simulink model "UNIFIER1"  (R2023b)
settings: Solver=ode1  StartTime=0.0  StopTime=t_sim  FixedStep=1/500  RelTol=1e-3
values from neighbouring files (symbols this model uses):
  b = 20.11467    [UNIFIERLanding_20240613_190735.mat]    (also in UNIFIER_LOAD.m; UNIFIER_LOADsim.m; UNIFIER_trim_out_20240612_032607.mat)
  c = 1.43676    [UNIFIERLanding_20240613_190735.mat]    (also in UNIFIER_LOAD.m; UNIFIER_LOADsim.m; UNIFIER_trim_out_20240612_032607.mat)
  DEP_INTEG_IC = 117.49388    [UNIFIER_LOAD.m]    (also in UNIFIER_LOADsim.m; UNIFIER_trim_out_20240612_032607.mat)
  dp_DEP =     [UNIFIERLanding_20240613_190735.mat]    (also in UNIFIER_trim_out_20240612_032607.mat)
  dp_FUSE_FIN =     [UNIFIER_trim_out_20240612_032607.mat]
  dp_HTU =     [UNIFIERLanding_20240613_190735.mat]    (also in UNIFIER_trim_out_20240612_032607.mat)
  dp_VTAIL =     [UNIFIER_trim_out_20240612_032607.mat]
  dp_VTAIL_INDUCED =     [UNIFIER_trim_out_20240612_032607.mat]
  dp_WING_root =     [UNIFIER_trim_out_20240612_032607.mat]
  dp_WING_tip =     [UNIFIER_trim_out_20240612_032607.mat]
  dumax = [1.0471975512 1.0471975512 1.0471975512 0.174532925199 2 2 2]    [UNIFIERLanding_20240613_190735.mat]
  Euler0 = xstar(7:9)'    [UNIFIER_6DOFsim_init.m]    (also in UNIFIER_LOAD.m = [0, 0, 0]; UNIFIER_LOADsim.m; UNIFIER_trim_out_20240612_032607.mat = [3.43106170069e-06 0.0515008506278 -2.79252663434])
  ground_alt = 0    [UNIFIER_LOAD.m]    (also in UNIFIER_LOADsim.m; UNIFIER_trim_out_20240612_032607.mat)
  m = 7057    [UNIFIERLanding_20240613_190735.mat]    (also in UNIFIER_LOAD.m; UNIFIER_LOADsim.m; UNIFIER_trim_out_20240612_032607.mat)
  omegab0 = xstar(10:12)'    [UNIFIER_6DOFsim_init.m]    (also in UNIFIER_LOAD.m = [0,0,0]; UNIFIER_LOADsim.m; UNIFIER_trim_out_20240612_032607.mat = [0 0 0])
  S = 29.98388    [UNIFIERLanding_20240613_190735.mat]    (also in UNIFIER_LOAD.m; UNIFIER_LOADsim.m; UNIFIER_trim_out_20240612_032607.mat)
  sensor_delay_steps = 5    [UNIFIER_LOAD.m]    (also in UNIFIER_LOADsim.m; UNIFIER_trim_out_20240612_032607.mat)
  solution =     [UNIFIERLanding_20240613_190735.mat]
  u1_0 = [ustar(1), -1*ustar(1), ustar(3)-ustar(2), ustar(3)+ustar(2), ustar(4), ustar(4)]    [UNIFIER_6DOFsim_init.m]    (also in UNIFIER_LOAD.m = [2.1112539e-05, -2.1112539e-05, -0.085004635, -0.084972650, ; UNIFIER_LOADsim.m = [2.1112539e-05, -2.1112539e-05, -0.085004635, -0.084972650, ; UNIFIER_trim_out_20240612_032607.mat = [2.1112539e-05 -2.1112539e-05 -0.085004635 -0.08497265 0.197)
  u2_0 = ones(1,12) .* ustar(5)    [UNIFIER_6DOFsim_init.m]    (also in UNIFIER_LOAD.m = ones(1,12) .* 0.4252; UNIFIER_LOADsim.m = ones(1,12) .* 0.4252; UNIFIER_trim_out_20240612_032607.mat = [0.4252 0.4252 0.4252 0.4252 0.4252 0.4252 0.4252 0.4252 0.4)
  u3_0 = ustar(7)    [UNIFIER_6DOFsim_init.m]    (also in UNIFIER_LOAD.m = 0.089689; UNIFIER_LOADsim.m = 0.089689; UNIFIER_trim_out_20240612_032607.mat = 0.089689)
  u4_0 = 0    [UNIFIER_6DOFsim_init.m]    (also in UNIFIER_LOAD.m; UNIFIER_LOADsim.m; UNIFIER_trim_out_20240612_032607.mat)
  u_trim = ustar    [UNIFIER_6DOFsim_init.m]    (also in UNIFIER_LOAD.m = [0.0; UNIFIER_LOADsim.m)
  umax = [0.436332312999 0.523598775598 0.523598775598 0.436332312999 1 1 1]    [UNIFIERLanding_20240613_190735.mat]    (also in UNIFIER_trim_out_20240612_032607.mat)
  umin = [-0.436332312999 -0.523598775598 -0.523598775598 0 0 -1 -0.5]    [UNIFIERLanding_20240613_190735.mat]    (also in UNIFIER_trim_out_20240612_032607.mat)
  Va = [72.7399985115 72.2978466179 70.3592089076 68.5755686022 67.5674222915 66.8967003826 65.8958642605 64.4243196248 62.667507398 61.0171213882 59.8601734245 59.2796795419 ... (250 elements, 250x1)]    [UNIFIERLanding_20240613_190735.mat]
  Vb0 = xstar(4:6)'    [UNIFIER_6DOFsim_init.m]    (also in UNIFIER_LOAD.m = [72.731047032614440, 0, 1.142307104518741]; UNIFIER_LOADsim.m; UNIFIER_trim_out_20240612_032607.mat = [52.6789583502 0 2.71559652634])
  vtail_dist_to_wing = 7.8070    (= 7.807)    [UNIFIER_LOAD.m]    (also in UNIFIER_LOADsim.m; UNIFIER_trim_out_20240612_032607.mat)
  vtail_nodes = [dp_VTAIL.Xs_LE;     dp_VTAIL.Ys_LE;     dp_VTAIL.Zs_LE]    [UNIFIER_LOAD.m]    (also in UNIFIER_LOADsim.m; UNIFIER_trim_out_20240612_032607.mat = [-16.4894695282 -2.83441376686 -2.73765826225 -16.1370849609)
  wing_nodes = [fliplr(dp_WING_tip.LE_Xs),fliplr(dp_WING_root.LE_Xs),dp_WING_root.LE_Xs,dp_WING_tip.LE_Xs;     fliplr(-dp_WING_tip.LE_Ys),fliplr(-dp_WING_root.LE_Ys),dp_WING_root.LE_Ys,dp_WING_tip.LE_Ys;     fliplr(dp_WING_tip.LE_Zs),fliplr(dp_WING_root.LE_Zs),dp_WING_root.LE_Zs,dp_WING_tip.LE_Zs]    [UNIFIER_LOAD.m]    (also in UNIFIER_LOADsim.m; UNIFIER_trim_out_20240612_032607.mat = [-7.70795631409 -9.67500019073 -0.98178178072 -7.66801691055)
  Xe0 = xstar(1:3)'    [UNIFIER_6DOFsim_init.m]    (also in UNIFIER_LOAD.m = [0,0,-1219]; UNIFIER_LOADsim.m; UNIFIER_trim_out_20240612_032607.mat = [0 0 -1100])
  xyz_cg = [-8.09 0 -0.2]    [UNIFIERLanding_20240613_190735.mat]    (also in UNIFIER_LOAD.m = [-8.09,0,-0.2]; UNIFIER_LOADsim.m = [-8.09,0,-0.2]; UNIFIER_trim_out_20240612_032607.mat)
  xyz_DEP = [-6.9629998 -10.05 -0.90899998 -6.921 -8.4499998 -0.792 -6.8660002 -6.8499999 -0.82300001 -6.8099999 -5.25 -0.85000002 ... (36 elements, 3x12)]    [UNIFIERLanding_20240613_190735.mat]    (also in UNIFIER_LOAD.m = [ -6.9629998	-6.9210000	-6.8660002	-6.8099999	-6.7540002	-6.; UNIFIER_LOADsim.m = [ -6.9629998	-6.9210000	-6.8660002	-6.8099999	-6.7540002	-6.; UNIFIER_trim_out_20240612_032607.mat)
undefined symbols (not defined in the file or in its folder): Earth, F, MIL, WGS84
libraries: simulink_extras x22, aerolibactuator x16, dspnetwork x15, sharedutil x14, sharedtransform x7, aerolibtransform2 x5, slpidlib x5, simulink x5, aerolibwind2 x4, matrix_library x1, shared6dof x1, aerolibatmos2 x1
(part 2 of 5)

== system UNIFIER1/FCC/Altitude Control ==
  note: swtich criteria:
      | 0 = real input
      | 1 = test (step) input
  Ze : Inport
  theta : Inport  Port=2
  q : Inport  Port=3
  Xe : Inport  Port=4
  1-D Lookup Table : Lookup_n-D  NumberOfTableDimensions=1  BreakpointsForDimension1=solution.X(:,1)  Table=solution.X(:,2)  InternalRulePriority=Speed  RndMeth=Simplest
  Bus Creator : BusCreator  Inputs=4
  Constant : Constant  Value=0
  Constant1 : Constant  Value=0
  Constant2 : Constant  Value=0
  Degrees to Radians : simulink_extras/Transformations/Degrees to Radians
  Degrees to Radians1 : simulink_extras/Transformations/Degrees to Radians
  PID_alt : slpidlib/PID Controller  Controller=PID  Form=Parallel  TimeDomain=Continuous-time  UseExternalTs=off  SampleTime=-1  IntegratorMethod=Forward Euler  FilterMethod=Forward Euler  ControllerParametersSource=internal  P=-0.003  I=-0.00025  UseKiTs=off  D=0  N=100  UseFilter=on  TunerSelectOption=Frequency Response Based  InitialConditionSource=internal  InitialConditionForIntegrator=0  InitialConditionForFilter=0  DifferentiatorICPrevScaledInput=0  ExternalReset=none  TrackingMode=off  Kt=1  LimitOutput=off  SatLimitsSource=internal  UpperSaturationLimit=inf  LowerSaturationLimit=-inf  LinearizeAsGain=on  AntiWindupMode=none  Kb=1  LimitIntegrator=off  UpperIntegratorSaturationLimit=inf  LowerIntegratorSaturationLimit=-inf  POutMin=[]  POutMax=[]  IOutMin=[]  IOutMax=[]  DOutMin=[]  DOutMax=[]  NOutMin=[]  NOutMax=[]  SumOutMin=[]  SumOutMax=[]  SaturationOutMin=[]  SaturationOutMax=[]  PParamMin=[]  PParamMax=[]  IParamMin=[]  IParamMax=[]  DParamMin=[]  DParamMax=[]  NParamMin=[]  NParamMax=[]  KbParamMin=[]  KbParamMax=[]  KtParamMin=[]  KtParamMax=[]  KbOutMin=[]  KbOutMax=[]  KtOutMin=[]  KtOutMax=[]  IntegratorOutMin=[]  IntegratorOutMax=[]  FilterOutMin=[]  FilterOutMax=[]  SumI1OutMin=[]  SumI1OutMax=[]  SumI2OutMin=[]  SumI2OutMax=[]  SumI3OutMin=[]  SumI3OutMax=[]  SumI4OutMin=[]  SumI4OutMax=[]  SumDOutMin=[]  SumDOutMax=[]  DifferentiatorOutMin=[]  DifferentiatorOutMax=[]  FilterDiffOutCoefMin=[]  FilterDiffOutCoefMax=[]  ReciprocalOutMin=[]  ReciprocalOutMax=[]  SumDenOutMin=[]  SumDenOutMax=[]  SumNumOutMin=[]  SumNumOutMax=[]  DivideOutMin=[]  DivideOutMax=[]  UdiffTsProdOutMin=[]  UdiffTsProdOutMax=[]  NTsProdOutMin=[]  NTsProdOutMax=[]  UintegralTsProdOutMin=[]  UintegralTsProdOutMax=[]  UngainTsProdOutMin=[]  UngainTsProdOutMax=[]  ClampingZeroOutDataTypeStr=Inherit: Inherit via back propagation  ClampingZeroOutMin=[]  ClampingZeroOutMax=[]  FilterDenConstantOutDataTypeStr=Inherit: Inherit via back propagation  FilterDenConstantOutMin=[]  FilterDenConstantOutMax=[]  PCopyOutDataTypeStr=Inherit: Inherit via back propagation  PCopyOutMin=[]  PCopyOutMax=[]  NCopyOutDataTypeStr=Inherit: Inherit via back propagation  NCopyOutMin=[]  NCopyOutMax=[]  IntegratorContinuousStateAttributes=''  IntegratorStateMustResolveToSignalObject=off  IntegratorRTWStateStorageClass=Auto  FilterContinuousStateAttributes=''  FilterStateMustResolveToSignalObject=off  FilterRTWStateStorageClass=Auto  ParallelPVariant=InternalParameters  IdealPVariant=Disabled  IVariant=InternalParameters  DVariant=InternalParameters  IntegratorVariant=Continuous  SatVariant=Disabled  AWVariant=Passthrough  PCopyVariant=Disabled  TRVariant=Disabled  FdbkBlocksVariant=Forward  IdealPFdbkVariant=Disabled  SatFdbkVariant=Disabled  DerivativeFilterVariant=ContFilter  NVariant=InternalParameters  NCopyVariant=Disabled  FilterICVariant=InternalICsFilter  IntegratorICVariant=InternalICs  ExternalResetVariant=Disabled  TRSumVariant=Passthrough  SumFdbkVariant=Disabled  SumVariant=Sum_PID  TsampFilterVariant=InternalTs  TsampNgainVariant=Passthrough  TsampIntegralVariant=Disabled_SignalSpec  ExternalSaturationOutDataTypeStr=Inherit: Same as second input
  PID_q : slpidlib/PID Controller  Controller=PID  Form=Parallel  TimeDomain=Continuous-time  UseExternalTs=off  SampleTime=-1  IntegratorMethod=Forward Euler  FilterMethod=Forward Euler  ControllerParametersSource=internal  P=-5  I=-50  UseKiTs=off  D=-0.1  N=100  UseFilter=on  TunerSelectOption=Transfer Function Based (PID Tuner App)  InitialConditionSource=internal  InitialConditionForIntegrator=0  InitialConditionForFilter=0  DifferentiatorICPrevScaledInput=0  ExternalReset=none  TrackingMode=off  Kt=1  LimitOutput=off  SatLimitsSource=internal  UpperSaturationLimit=inf  LowerSaturationLimit=-inf  LinearizeAsGain=on  AntiWindupMode=none  Kb=1  LimitIntegrator=off  UpperIntegratorSaturationLimit=inf  LowerIntegratorSaturationLimit=-inf  POutMin=[]  POutMax=[]  IOutMin=[]  IOutMax=[]  DOutMin=[]  DOutMax=[]  NOutMin=[]  NOutMax=[]  SumOutMin=[]  SumOutMax=[]  SaturationOutMin=[]  SaturationOutMax=[]  PParamMin=[]  PParamMax=[]  IParamMin=[]  IParamMax=[]  DParamMin=[]  DParamMax=[]  NParamMin=[]  NParamMax=[]  KbParamMin=[]  KbParamMax=[]  KtParamMin=[]  KtParamMax=[]  KbOutMin=[]  KbOutMax=[]  KtOutMin=[]  KtOutMax=[]  IntegratorOutMin=[]  IntegratorOutMax=[]  FilterOutMin=[]  FilterOutMax=[]  SumI1OutMin=[]  SumI1OutMax=[]  SumI2OutMin=[]  SumI2OutMax=[]  SumI3OutMin=[]  SumI3OutMax=[]  SumI4OutMin=[]  SumI4OutMax=[]  SumDOutMin=[]  SumDOutMax=[]  DifferentiatorOutMin=[]  DifferentiatorOutMax=[]  FilterDiffOutCoefMin=[]  FilterDiffOutCoefMax=[]  ReciprocalOutMin=[]  ReciprocalOutMax=[]  SumDenOutMin=[]  SumDenOutMax=[]  SumNumOutMin=[]  SumNumOutMax=[]  DivideOutMin=[]  DivideOutMax=[]  UdiffTsProdOutMin=[]  UdiffTsProdOutMax=[]  NTsProdOutMin=[]  NTsProdOutMax=[]  UintegralTsProdOutMin=[]  UintegralTsProdOutMax=[]  UngainTsProdOutMin=[]  UngainTsProdOutMax=[]  ClampingZeroOutDataTypeStr=Inherit: Inherit via back propagation  ClampingZeroOutMin=[]  ClampingZeroOutMax=[]  FilterDenConstantOutDataTypeStr=Inherit: Inherit via back propagation  FilterDenConstantOutMin=[]  FilterDenConstantOutMax=[]  PCopyOutDataTypeStr=Inherit: Inherit via back propagation  PCopyOutMin=[]  PCopyOutMax=[]  NCopyOutDataTypeStr=Inherit: Inherit via back propagation  NCopyOutMin=[]  NCopyOutMax=[]  IntegratorContinuousStateAttributes=''  IntegratorStateMustResolveToSignalObject=off  IntegratorRTWStateStorageClass=Auto  FilterContinuousStateAttributes=''  FilterStateMustResolveToSignalObject=off  FilterRTWStateStorageClass=Auto  ParallelPVariant=InternalParameters  IdealPVariant=Disabled  IVariant=InternalParameters  DVariant=InternalParameters  IntegratorVariant=Continuous  SatVariant=Disabled  AWVariant=Passthrough  PCopyVariant=Disabled  TRVariant=Disabled  FdbkBlocksVariant=Forward  IdealPFdbkVariant=Disabled  SatFdbkVariant=Disabled  DerivativeFilterVariant=ContFilter  NVariant=InternalParameters  NCopyVariant=Disabled  FilterICVariant=InternalICsFilter  IntegratorICVariant=InternalICs  ExternalResetVariant=Disabled  TRSumVariant=Passthrough  SumFdbkVariant=Disabled  SumVariant=Sum_PID  TsampFilterVariant=InternalTs  TsampNgainVariant=Passthrough  TsampIntegralVariant=Disabled_SignalSpec  ExternalSaturationOutDataTypeStr=Inherit: Same as second input
  PID_theta : slpidlib/PID Controller  Controller=PID  Form=Parallel  TimeDomain=Continuous-time  UseExternalTs=off  SampleTime=-1  IntegratorMethod=Forward Euler  FilterMethod=Forward Euler  ControllerParametersSource=internal  P=2.25  I=0  UseKiTs=off  D=0  N=100  UseFilter=on  TunerSelectOption=Transfer Function Based (PID Tuner App)  InitialConditionSource=internal  InitialConditionForIntegrator=0  InitialConditionForFilter=0  DifferentiatorICPrevScaledInput=0  ExternalReset=none  TrackingMode=off  Kt=1  LimitOutput=off  SatLimitsSource=internal  UpperSaturationLimit=inf  LowerSaturationLimit=-inf  LinearizeAsGain=on  AntiWindupMode=none  Kb=1  LimitIntegrator=off  UpperIntegratorSaturationLimit=inf  LowerIntegratorSaturationLimit=-inf  POutMin=[]  POutMax=[]  IOutMin=[]  IOutMax=[]  DOutMin=[]  DOutMax=[]  NOutMin=[]  NOutMax=[]  SumOutMin=[]  SumOutMax=[]  SaturationOutMin=[]  SaturationOutMax=[]  PParamMin=[]  PParamMax=[]  IParamMin=[]  IParamMax=[]  DParamMin=[]  DParamMax=[]  NParamMin=[]  NParamMax=[]  KbParamMin=[]  KbParamMax=[]  KtParamMin=[]  KtParamMax=[]  KbOutMin=[]  KbOutMax=[]  KtOutMin=[]  KtOutMax=[]  IntegratorOutMin=[]  IntegratorOutMax=[]  FilterOutMin=[]  FilterOutMax=[]  SumI1OutMin=[]  SumI1OutMax=[]  SumI2OutMin=[]  SumI2OutMax=[]  SumI3OutMin=[]  SumI3OutMax=[]  SumI4OutMin=[]  SumI4OutMax=[]  SumDOutMin=[]  SumDOutMax=[]  DifferentiatorOutMin=[]  DifferentiatorOutMax=[]  FilterDiffOutCoefMin=[]  FilterDiffOutCoefMax=[]  ReciprocalOutMin=[]  ReciprocalOutMax=[]  SumDenOutMin=[]  SumDenOutMax=[]  SumNumOutMin=[]  SumNumOutMax=[]  DivideOutMin=[]  DivideOutMax=[]  UdiffTsProdOutMin=[]  UdiffTsProdOutMax=[]  NTsProdOutMin=[]  NTsProdOutMax=[]  UintegralTsProdOutMin=[]  UintegralTsProdOutMax=[]  UngainTsProdOutMin=[]  UngainTsProdOutMax=[]  ClampingZeroOutDataTypeStr=Inherit: Inherit via back propagation  ClampingZeroOutMin=[]  ClampingZeroOutMax=[]  FilterDenConstantOutDataTypeStr=Inherit: Inherit via back propagation  FilterDenConstantOutMin=[]  FilterDenConstantOutMax=[]  PCopyOutDataTypeStr=Inherit: Inherit via back propagation  PCopyOutMin=[]  PCopyOutMax=[]  NCopyOutDataTypeStr=Inherit: Inherit via back propagation  NCopyOutMin=[]  NCopyOutMax=[]  IntegratorContinuousStateAttributes=''  IntegratorStateMustResolveToSignalObject=off  IntegratorRTWStateStorageClass=Auto  FilterContinuousStateAttributes=''  FilterStateMustResolveToSignalObject=off  FilterRTWStateStorageClass=Auto  ParallelPVariant=InternalParameters  IdealPVariant=Disabled  IVariant=InternalParameters  DVariant=InternalParameters  IntegratorVariant=Continuous  SatVariant=Disabled  AWVariant=Passthrough  PCopyVariant=Disabled  TRVariant=Disabled  FdbkBlocksVariant=Forward  IdealPFdbkVariant=Disabled  SatFdbkVariant=Disabled  DerivativeFilterVariant=ContFilter  NVariant=InternalParameters  NCopyVariant=Disabled  FilterICVariant=InternalICsFilter  IntegratorICVariant=InternalICs  ExternalResetVariant=Disabled  TRSumVariant=Passthrough  SumFdbkVariant=Disabled  SumVariant=Sum_PID  TsampFilterVariant=InternalTs  TsampNgainVariant=Passthrough  TsampIntegralVariant=Disabled_SignalSpec  ExternalSaturationOutDataTypeStr=Inherit: Same as second input
  Saturation1 : Saturate  UpperLimit=0  LowerLimit=-inf
  Sum : Sum  Inputs=|+-
  Sum3 : Sum  Inputs=|+-
  Sum4 : Sum  Inputs=|+-
  Switch : Switch  Criteria=u2 > Threshold  SaturateOnIntegerOverflow=off  InputSameDT=off
  Switch1 : Switch  Criteria=u2 > Threshold  SaturateOnIntegerOverflow=off  InputSameDT=off
  Switch2 : Switch  Criteria=u2 > Threshold  SaturateOnIntegerOverflow=off  InputSameDT=off
  Ze_step : Step  Time=40  Before=-1219  After=-1269  SampleTime=0
  q_step : Step  Time=5  After=0  SampleTime=0
  theta_step : Step  Time=7  Before=0.9  After=2  SampleTime=0
  elev : Outport
  scopeout : Outport  Port=2
  wires:
  Ze/1 -> Sum/2
  Sum/1 -> PID_alt/1
  q/1 -> Sum4/2
  theta/1 -> Sum3/2
  PID_q/1 -> elev/1, Bus Creator/4  "elev_cmd"
  Sum4/1 -> PID_q/1
  Sum3/1 -> PID_theta/1
  theta_step/1 -> Degrees to Radians/1
  q_step/1 -> Degrees to Radians1/1
  Switch1/1 -> Bus Creator/2, Sum3/1  "theta_cmd"
  Degrees to Radians/1 -> Switch1/1
  Xe/1 -> 1-D Lookup Table/1
  1-D Lookup Table/1 -> Saturation1/1
  Switch/1 -> Sum/1, Bus Creator/1  "Ze_ref"
  Switch2/1 -> Bus Creator/3, Sum4/1  "q_cmd"
  Bus Creator/1 -> scopeout/1
  Ze_step/1 -> Switch/1
  Degrees to Radians1/1 -> Switch2/1
  Saturation1/1 -> Switch/3
  Constant/1 -> Switch/2
  PID_alt/1 -> Switch1/3
  PID_theta/1 -> Switch2/3
  Constant2/1 -> Switch2/2
  Constant1/1 -> Switch1/2

== system UNIFIER1/FCC/Ganging ==
  u_ganged : Inport
  Constant : Constant  Value=0
  Demux : Demux  Outputs=7
  For Each Subsystem : Subsystem  TreatAsAtomicUnit=on
  Mux : Mux  Inputs=2
  Mux1 : Mux  Inputs=2
  Mux2 : Mux  Inputs=2
  Mux3 : Mux  Inputs=[6 12 1 1]
  Mux4 : Mux  Inputs=3
  Unary Minus : UnaryMinus
  V-tail mixing : Subsystem
  zeta : Constant  Value=[-1, -0.8, -0.4, -0.2, -0.1, 0, 0, 0.1, 0.2, 0.4, 0.8, 1]
  u : Outport
  wires:
  u_ganged/1 -> Demux/1
  Mux3/1 -> u/1
  Demux/1 -> Mux/1, Unary Minus/1  "ail"
  Unary Minus/1 -> Mux/2
  V-tail mixing/1(rudL) -> Mux1/1
  V-tail mixing/2(rudR) -> Mux1/2
  Demux/4 -> Mux2/2, Mux2/1  "flap"
  Demux/7 -> Mux3/3  "u3"
  Mux/1 -> Mux4/1  "ail"
  Mux1/1 -> Mux4/2  "rud"
  Mux2/1 -> Mux4/3  "flap"
  Demux/5 -> For Each Subsystem/2(DEP_col)  "DEP_col"
  Demux/6 -> For Each Subsystem/3(DEP_slope)  "DEP_slp"
  For Each Subsystem/1(Out1) -> Mux3/2  "u2"
  Mux4/1 -> Mux3/1  "u1"
  Constant/1 -> Mux3/4  "u4"
  zeta/1 -> For Each Subsystem/1(zeta)
  Demux/2 -> V-tail mixing/1(rud)  "rud"
  Demux/3 -> V-tail mixing/2(elev)  "elev"

== system UNIFIER1/FCC/Manual ==
  aileron : Inport
  elevator : Inport  Port=2
  rudder : Inport  Port=3
  throttle : Inport  Port=4
  Constant : Constant  Value=deg2rad(10)
  Constant1 : Constant
  Constant2 : Constant  Value=0
  Dead Zone : DeadZone  LowerValue=-0.1  UpperValue=0.1
  Dead Zone1 : DeadZone  LowerValue=-0.1  UpperValue=0.1
  Dead Zone2 : DeadZone  LowerValue=-0.1  UpperValue=0.1
  Gain : Gain  Gain=deg2rad(20)
  Gain1 : Gain  Gain=-deg2rad(30)
  Gain2 : Gain  Gain=deg2rad(15)
  Gain3 : Gain  Gain=1.5
  Mux : Mux  Inputs=6
  Mux1 : Mux  Inputs=12
  Saturation : Saturate  UpperLimit=deg2rad(30)  LowerLimit=-deg2rad(30)
  Saturation1 : Saturate  UpperLimit=deg2rad(30)  LowerLimit=-deg2rad(30)
  Saturation2 : Saturate  UpperLimit=deg2rad(20)  LowerLimit=-deg2rad(20)
  Saturation3 : Saturate  UpperLimit=deg2rad(20)  LowerLimit=-deg2rad(20)
  Sum : Sum  Inputs=|++
  Sum1 : Sum  Inputs=|++
  Unary Minus : UnaryMinus
  Unary Minus1 : UnaryMinus
  Vector Concatenate : Concatenate  NumInputs=4
  u : Outport
  wires:
  aileron/1 -> Dead Zone/1
  elevator/1 -> Dead Zone1/1
  Unary Minus/1 -> Saturation2/1
  Gain/1 -> Unary Minus/1, Saturation3/1
  Gain1/1 -> Sum1/1, Sum/1
  Sum1/1 -> Saturation1/1
  Saturation/1 -> Mux/3
  Sum/1 -> Saturation/1
  Saturation1/1 -> Mux/4
  rudder/1 -> Dead Zone2/1
  Gain2/1 -> Sum1/2, Unary Minus1/1
  Saturation2/1 -> Mux/2
  Saturation3/1 -> Mux/1
  Mux/1 -> Vector Concatenate/1
  Vector Concatenate/1 -> u/1
  Constant/1 -> Mux/6, Mux/5
  Mux1/1 -> Vector Concatenate/2
  Unary Minus1/1 -> Sum/2
  Constant1/1 -> Vector Concatenate/4
  Dead Zone/1 -> Gain/1
  Dead Zone1/1 -> Gain1/1
  Dead Zone2/1 -> Gain2/1
  throttle/1 -> Gain3/1, Mux1/1, Mux1/2, Mux1/3, Mux1/12, Mux1/11, Mux1/10
  Constant2/1 -> Mux1/4, Mux1/5, Mux1/9, Mux1/8, Mux1/7, Mux1/6
  Gain3/1 -> Vector Concatenate/3

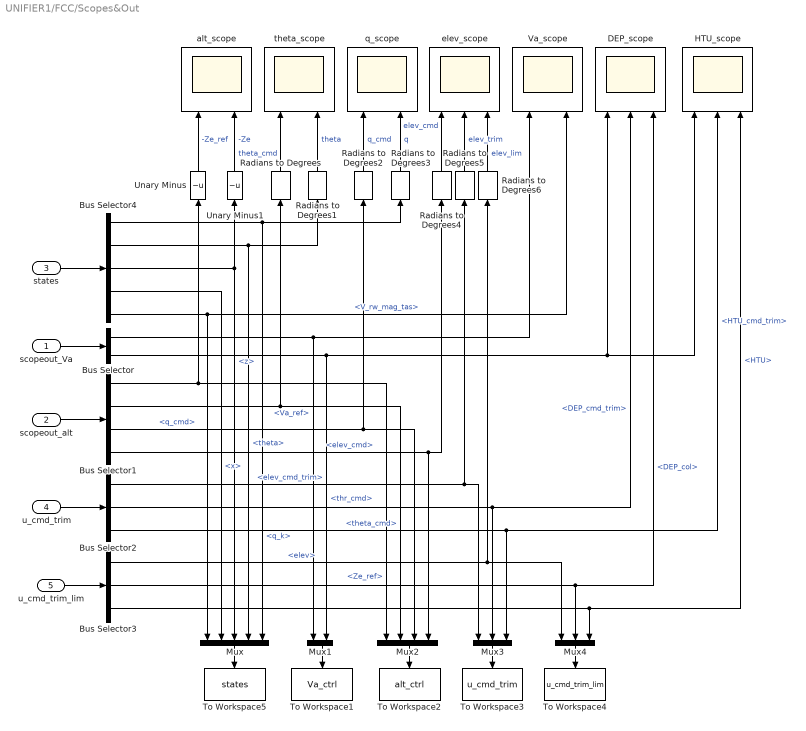
== system UNIFIER1/FCC/Scopes&Out ==
  scopeout_Va : Inport
  scopeout_alt : Inport  Port=2
  states : Inport  Port=3
  u_cmd_trim : Inport  Port=4
  u_cmd_trim_lim : Inport  Port=5
  Bus Selector : BusSelector  OutputSignals=Va_ref,thr_cmd
  Bus Selector1 : BusSelector  OutputSignals=Ze_ref,theta_cmd,q_cmd,elev_cmd
  Bus Selector2 : BusSelector  OutputSignals=elev_cmd_trim,DEP_cmd_trim,HTU_cmd_trim
  Bus Selector3 : BusSelector  OutputSignals=elev,DEP_col,HTU
  Bus Selector4 : BusSelector  OutputSignals=q_k,theta,z,x,V_rw_mag_tas
  DEP_scope : Scope  NumInputPorts=3
  HTU_scope : Scope  NumInputPorts=3
  Mux : Mux  Inputs=5
  Mux1 : Mux  Inputs=2
  Mux2 : Mux
  Mux3 : Mux  Inputs=3
  Mux4 : Mux  Inputs=3
  Radians to Degrees{,1..6} (7 alike) : simulink_extras/Transformations/Radians to Degrees
  To Workspace1 : ToWorkspace  VariableName=Va_ctrl  SampleTime=-1
  To Workspace2 : ToWorkspace  VariableName=alt_ctrl  SampleTime=-1
  To Workspace3 : ToWorkspace  VariableName=u_cmd_trim  SampleTime=-1
  To Workspace4 : ToWorkspace  VariableName=u_cmd_trim_lim  SampleTime=-1
  To Workspace5 : ToWorkspace  VariableName=states  SampleTime=-1
  Unary Minus : UnaryMinus
  Unary Minus1 : UnaryMinus
  Va_scope : Scope  NumInputPorts=2
  alt_scope : Scope  NumInputPorts=2
  elev_scope : Scope  NumInputPorts=3
  q_scope : Scope  NumInputPorts=2
  theta_scope : Scope  NumInputPorts=2
  wires:
  scopeout_Va/1 -> Bus Selector/1
  scopeout_alt/1 -> Bus Selector1/1
  u_cmd_trim/1 -> Bus Selector2/1
  u_cmd_trim_lim/1 -> Bus Selector3/1
  Bus Selector3/2 -> Mux4/2, DEP_scope/3  "<DEP_col>"
  Bus Selector3/3 -> Mux4/3, HTU_scope/3  "<HTU>"
  Bus Selector/2 -> HTU_scope/1, DEP_scope/1, Mux1/2  "<thr_cmd>"
  Bus Selector/1 -> Va_scope/1, Mux1/1  "<Va_ref>"
  states/1 -> Bus Selector4/1
  Bus Selector2/2 -> DEP_scope/2, Mux3/2  "<DEP_cmd_trim>"
  Bus Selector2/3 -> Mux3/3, HTU_scope/2  "<HTU_cmd_trim>"
  Bus Selector1/1 -> Mux2/1, Unary Minus/1  "<Ze_ref>"
  Unary Minus/1 -> alt_scope/1  "-Ze_ref"
  Unary Minus1/1 -> alt_scope/2  "-Ze"
  Radians to Degrees/1 -> theta_scope/1  "theta_cmd"
  Radians to Degrees1/1 -> theta_scope/2  "theta"
  Bus Selector4/2 -> Radians to Degrees1/1, Mux/4  "<theta>"
  Bus Selector1/2 -> Mux2/2, Radians to Degrees/1  "<theta_cmd>"
  Radians to Degrees2/1 -> q_scope/1  "q_cmd"
  Radians to Degrees3/1 -> q_scope/2  "q"
  Bus Selector4/1 -> Radians to Degrees3/1, Mux/5  "<q_k>"
  Bus Selector1/3 -> Mux2/3, Radians to Degrees2/1  "<q_cmd>"
  Radians to Degrees4/1 -> elev_scope/1  "elev_cmd"
  Radians to Degrees5/1 -> elev_scope/2  "elev_trim"
  Radians to Degrees6/1 -> elev_scope/3  "elev_lim"
  Bus Selector1/4 -> Mux2/4, Radians to Degrees4/1  "<elev_cmd>"
  Bus Selector2/1 -> Mux3/1, Radians to Degrees5/1  "<elev_cmd_trim>"
  Bus Selector3/1 -> Mux4/1, Radians to Degrees6/1  "<elev>"
  Bus Selector4/5 -> Va_scope/2, Mux/1  "<V_rw_mag_tas>"
  Bus Selector4/3 -> Mux/3, Unary Minus1/1  "<z>"
  Bus Selector4/4 -> Mux/2  "<x>"
  Mux/1 -> To Workspace5/1
  Mux1/1 -> To Workspace1/1
  Mux2/1 -> To Workspace2/1
  Mux3/1 -> To Workspace3/1
  Mux4/1 -> To Workspace4/1

== system UNIFIER1/PACER/Output to Console ==
  note: Note: Constant in green block
      |           can be changed on the fly.
  data to console : Inport
  Enable : EnablePort
  Number of sim steps to skip : Constant  Value=1000
  S-Function : S-Function  FunctionName=sfun_output_to_console  Parameters='[tSimElapsed, tWallElapsed, absTimeErr (s)]: '  SFunctionDeploymentMode=off  EnableBusSupport=off
  skip every N'th : Display
  wires:
  Number of sim steps to skip/1 -> S-Function/1, skip every N'th/1
  data to console/1 -> S-Function/2

== system UNIFIER1/PACER/Subsystem ==

== system UNIFIER1/PACER/soft real time subsystem ==
  note: What is elapsed real
      | wall-clock time?
  note: What is elapsed
      | simulation time?
  note: Sleep this amount
      | to advance sim time
      | same as wall time
  note: Typically a simple (enough) simulation will fun faster than
      | wall-clock time. This means it's possible for Simulink to
      | simulate, say, 10 seconds in perhps 0.1 or 1 seconds of real
      | wall-clock time.
      |
      | So the challenge is this: how much pause should be inserted
      | every so often to cause the simulation time to advance at
      | the same average rate as real wall-clock time?
      |
      | Using total elapsed time as an absolute reference, this
      | sleep duration will ensure no drift accumulation:
      |
      |      t_sleep = t_elapsed_sim_time - t_elapsed_wall_clock_time
      |
      | Pace error and Sleep() or usleep() resolution is system dependent
      | and likely around 10ms on Windows machines. Better on linux.
      |
      | Marc Compere
      | comperem@gmail.com
      | created : 28 May 2018
      | modified: 29 May 2018
  Constant : Constant  Value=0
  Display : Display
  MinMax : MinMax  Function=max  Inputs=2
  S-Function : S-Function  FunctionName=sfun_sleep  Parameters=t_sample  SFunctionDeploymentMode=off  EnableBusSupport=off
  Sum : Sum  Inputs=|+-
  get elapsed wall-clock time : Subsystem
  s --> ms : Gain  Gain=1000
  simulation time (s) : Clock
  t_elapsed_wall_clock (s) : Outport
  pace error (s) : Outport  Port=2
  wires:
  simulation time (s)/1 -> Sum/1
  Constant/1 -> MinMax/2
  get elapsed wall-clock time/1(t_wall_clock_elapsed (s)) -> t_elapsed_wall_clock (s)/1, Sum/2
  Sum/1 -> Display/1, MinMax/1  "pace error (s)"
  MinMax/1 -> pace error (s)/1, s --> ms/1
  s --> ms/1 -> S-Function/1  "sleep duration (ms)"

== system UNIFIER1/X_PLANE_VISUALS/DEPSpinning ==
  note: MAKE THE PUSHER PROP SPIN IN VISUALIZATION
  actf : Inport
  Constant2 : Constant  Value=0
  Constant3 : Constant  Value=10
  Memory1 : Memory  InheritSampleTime=on
  Product : Product
  Scope : Scope
  Sum : Sum  Inputs=|++
  Switch : Switch  Criteria=u2 > Threshold  Threshold=360  SaturateOnIntegerOverflow=off  InputSameDT=off
  angle : Outport
  wires:
  Sum/1 -> Switch/2, Switch/3
  Switch/1 -> angle/1, Memory1/1
  Memory1/1 -> Scope/1, Sum/2
  Product/1 -> Sum/1
  Constant2/1 -> Switch/1
  actf/1 -> Product/1
  Constant3/1 -> Product/2

== system UNIFIER1/X_PLANE_VISUALS/PusherSpinning ==
  note: MAKE THE PUSHER PROP SPIN IN VISUALIZATION
  actf : Inport
  Constant2 : Constant  Value=0
  Constant3 : Constant  Value=10
  Memory1 : Memory  InheritSampleTime=on
  Product : Product
  Scope : Scope
  Sum : Sum  Inputs=|++
  Switch : Switch  Criteria=u2 > Threshold  Threshold=360  SaturateOnIntegerOverflow=off  InputSameDT=off
  angle : Outport
  wires:
  Sum/1 -> Switch/2, Switch/3
  Switch/1 -> angle/1, Memory1/1
  Memory1/1 -> Scope/1, Sum/2
  Product/1 -> Sum/1
  Constant2/1 -> Switch/1
  actf/1 -> Product/1
  Constant3/1 -> Product/2

== system UNIFIER1/X_PLANE_VISUALS/Subsystem ==
  value : Inport
  Constant : Constant  Value=uint8(str)
  DREF : MATLAB Function  TreatAsAtomicUnit=on
  Data Type Conversion2 : DataTypeConversion  OutDataTypeStr=single  SaturateOnIntegerOverflow=off  RndMeth=Floor
  UDP Send1 : dspnetwork/UDP Send  remoteURL='127.0.0.1'  remotePort=49000  localURL='0.0.0.0'  localPortSource=Automatically determine  localPort=-1  sendBufferSize=8192  sampletime=-1  blockPlatform=[]  separateLengthPort=0
  wires:
  Data Type Conversion2/1 -> DREF/2(value)
  DREF/1(uint8_out) -> UDP Send1/1
  Constant/1 -> DREF/1(str)
  value/1 -> Data Type Conversion2/1

== system UNIFIER1/X_PLANE_VISUALS/Subsystem1 ==
  value : Inport
  Constant : Constant  Value=uint8(str)
  DREF : MATLAB Function  TreatAsAtomicUnit=on
  Data Type Conversion2 : DataTypeConversion  OutDataTypeStr=single  SaturateOnIntegerOverflow=off  RndMeth=Floor
  UDP Send1 : dspnetwork/UDP Send  remoteURL='127.0.0.1'  remotePort=49000  localURL='0.0.0.0'  localPortSource=Automatically determine  localPort=-1  sendBufferSize=8192  sampletime=-1  blockPlatform=[]  separateLengthPort=0
  wires:
  Data Type Conversion2/1 -> DREF/2(value)
  DREF/1(uint8_out) -> UDP Send1/1
  Constant/1 -> DREF/1(str)
  value/1 -> Data Type Conversion2/1

== system UNIFIER1/X_PLANE_VISUALS/Subsystem10 ==
  value : Inport
  Constant : Constant  Value=uint8(str)
  DREF : MATLAB Function  TreatAsAtomicUnit=on
  Data Type Conversion2 : DataTypeConversion  OutDataTypeStr=single  SaturateOnIntegerOverflow=off  RndMeth=Floor
  UDP Send1 : dspnetwork/UDP Send  remoteURL='127.0.0.1'  remotePort=49000  localURL='0.0.0.0'  localPortSource=Automatically determine  localPort=-1  sendBufferSize=8192  sampletime=-1  blockPlatform=[]  separateLengthPort=0
  wires:
  value/1 -> Data Type Conversion2/1
  Constant/1 -> DREF/1(str)
  DREF/1(uint8_out) -> UDP Send1/1
  Data Type Conversion2/1 -> DREF/2(value)

== system UNIFIER1/X_PLANE_VISUALS/Subsystem11 ==
  value : Inport
  Constant : Constant  Value=uint8(str)
  DREF : MATLAB Function  TreatAsAtomicUnit=on
  Data Type Conversion2 : DataTypeConversion  OutDataTypeStr=single  SaturateOnIntegerOverflow=off  RndMeth=Floor
  UDP Send1 : dspnetwork/UDP Send  remoteURL='127.0.0.1'  remotePort=49000  localURL='0.0.0.0'  localPortSource=Automatically determine  localPort=-1  sendBufferSize=8192  sampletime=-1  blockPlatform=[]  separateLengthPort=0
  wires:
  value/1 -> Data Type Conversion2/1
  Constant/1 -> DREF/1(str)
  DREF/1(uint8_out) -> UDP Send1/1
  Data Type Conversion2/1 -> DREF/2(value)

== system UNIFIER1/X_PLANE_VISUALS/Subsystem2 ==
  value : Inport
  Constant : Constant  Value=uint8(str)
  DREF : MATLAB Function  TreatAsAtomicUnit=on
  Data Type Conversion2 : DataTypeConversion  OutDataTypeStr=single  SaturateOnIntegerOverflow=off  RndMeth=Floor
  UDP Send1 : dspnetwork/UDP Send  remoteURL='127.0.0.1'  remotePort=49000  localURL='0.0.0.0'  localPortSource=Automatically determine  localPort=-1  sendBufferSize=8192  sampletime=-1  blockPlatform=[]  separateLengthPort=0
  wires:
  value/1 -> Data Type Conversion2/1
  Constant/1 -> DREF/1(str)
  DREF/1(uint8_out) -> UDP Send1/1
  Data Type Conversion2/1 -> DREF/2(value)

== system UNIFIER1/X_PLANE_VISUALS/Subsystem3 ==
  value : Inport
  Constant : Constant  Value=uint8(str)
  DREF : MATLAB Function  TreatAsAtomicUnit=on
  Data Type Conversion2 : DataTypeConversion  OutDataTypeStr=single  SaturateOnIntegerOverflow=off  RndMeth=Floor
  UDP Send1 : dspnetwork/UDP Send  remoteURL='127.0.0.1'  remotePort=49000  localURL='0.0.0.0'  localPortSource=Automatically determine  localPort=-1  sendBufferSize=8192  sampletime=-1  blockPlatform=[]  separateLengthPort=0
  wires:
  Data Type Conversion2/1 -> DREF/2(value)
  DREF/1(uint8_out) -> UDP Send1/1
  Constant/1 -> DREF/1(str)
  value/1 -> Data Type Conversion2/1

== system UNIFIER1/X_PLANE_VISUALS/Subsystem4 ==
  value : Inport
  Constant : Constant  Value=uint8(str)
  DREF : MATLAB Function  TreatAsAtomicUnit=on
  Data Type Conversion2 : DataTypeConversion  OutDataTypeStr=single  SaturateOnIntegerOverflow=off  RndMeth=Floor
  UDP Send1 : dspnetwork/UDP Send  remoteURL='127.0.0.1'  remotePort=49000  localURL='0.0.0.0'  localPortSource=Automatically determine  localPort=-1  sendBufferSize=8192  sampletime=-1  blockPlatform=[]  separateLengthPort=0
  wires:
  value/1 -> Data Type Conversion2/1
  Constant/1 -> DREF/1(str)
  DREF/1(uint8_out) -> UDP Send1/1
  Data Type Conversion2/1 -> DREF/2(value)

== system UNIFIER1/X_PLANE_VISUALS/Subsystem5 ==
  value : Inport
  Constant : Constant  Value=uint8(str)
  DREF : MATLAB Function  TreatAsAtomicUnit=on
  Data Type Conversion2 : DataTypeConversion  OutDataTypeStr=single  SaturateOnIntegerOverflow=off  RndMeth=Floor
  UDP Send1 : dspnetwork/UDP Send  remoteURL='127.0.0.1'  remotePort=49000  localURL='0.0.0.0'  localPortSource=Automatically determine  localPort=-1  sendBufferSize=8192  sampletime=-1  blockPlatform=[]  separateLengthPort=0
  wires:
  value/1 -> Data Type Conversion2/1
  Constant/1 -> DREF/1(str)
  DREF/1(uint8_out) -> UDP Send1/1
  Data Type Conversion2/1 -> DREF/2(value)

== system UNIFIER1/X_PLANE_VISUALS/Subsystem6 ==
  value : Inport
  Constant : Constant  Value=uint8(str)
  DREF : MATLAB Function  TreatAsAtomicUnit=on
  Data Type Conversion2 : DataTypeConversion  OutDataTypeStr=single  SaturateOnIntegerOverflow=off  RndMeth=Floor
  UDP Send1 : dspnetwork/UDP Send  remoteURL='127.0.0.1'  remotePort=49000  localURL='0.0.0.0'  localPortSource=Automatically determine  localPort=-1  sendBufferSize=8192  sampletime=-1  blockPlatform=[]  separateLengthPort=0
  wires:
  value/1 -> Data Type Conversion2/1
  Constant/1 -> DREF/1(str)
  DREF/1(uint8_out) -> UDP Send1/1
  Data Type Conversion2/1 -> DREF/2(value)

== system UNIFIER1/X_PLANE_VISUALS/Subsystem7 ==
  value : Inport
  Constant : Constant  Value=uint8(str)
  DREF : MATLAB Function  TreatAsAtomicUnit=on
  Data Type Conversion2 : DataTypeConversion  OutDataTypeStr=single  SaturateOnIntegerOverflow=off  RndMeth=Floor
  UDP Send1 : dspnetwork/UDP Send  remoteURL='127.0.0.1'  remotePort=49000  localURL='0.0.0.0'  localPortSource=Automatically determine  localPort=-1  sendBufferSize=8192  sampletime=-1  blockPlatform=[]  separateLengthPort=0
  wires:
  value/1 -> Data Type Conversion2/1
  Constant/1 -> DREF/1(str)
  DREF/1(uint8_out) -> UDP Send1/1
  Data Type Conversion2/1 -> DREF/2(value)

== system UNIFIER1/X_PLANE_VISUALS/Subsystem8 ==
  value : Inport
  Constant : Constant  Value=uint8(str)
  DREF : MATLAB Function  TreatAsAtomicUnit=on
  Data Type Conversion2 : DataTypeConversion  OutDataTypeStr=single  SaturateOnIntegerOverflow=off  RndMeth=Floor
  UDP Send1 : dspnetwork/UDP Send  remoteURL='127.0.0.1'  remotePort=49000  localURL='0.0.0.0'  localPortSource=Automatically determine  localPort=-1  sendBufferSize=8192  sampletime=-1  blockPlatform=[]  separateLengthPort=0
  wires:
  value/1 -> Data Type Conversion2/1
  Constant/1 -> DREF/1(str)
  DREF/1(uint8_out) -> UDP Send1/1
  Data Type Conversion2/1 -> DREF/2(value)

== system UNIFIER1/X_PLANE_VISUALS/Subsystem9 ==
  value : Inport
  Constant : Constant  Value=uint8(str)
  DREF : MATLAB Function  TreatAsAtomicUnit=on
  Data Type Conversion2 : DataTypeConversion  OutDataTypeStr=single  SaturateOnIntegerOverflow=off  RndMeth=Floor
  UDP Send1 : dspnetwork/UDP Send  remoteURL='127.0.0.1'  remotePort=49000  localURL='0.0.0.0'  localPortSource=Automatically determine  localPort=-1  sendBufferSize=8192  sampletime=-1  blockPlatform=[]  separateLengthPort=0
  wires:
  value/1 -> Data Type Conversion2/1
  Constant/1 -> DREF/1(str)
  DREF/1(uint8_out) -> UDP Send1/1
  Data Type Conversion2/1 -> DREF/2(value)

== system UNIFIER1/X_PLANE_VISUALS/override_flightcontrol  ==
  Trigger : TriggerPort  VariantControl=(inherit)  InitialTriggerSignalState=zero
  Constant : Constant
  Subsystem : Subsystem  mask{str='sim/operation/override/override_flightcontrol'}
      mask prompts: str "dref"
  wires:
  Constant/1 -> Subsystem/1(value)

== system UNIFIER1/X_PLANE_VISUALS/override_flightcontrol 1 ==
  Trigger : TriggerPort  VariantControl=(inherit)  InitialTriggerSignalState=zero
  Constant : Constant
  Subsystem : Subsystem  mask{str='sim/operation/override/override_control_surfaces'}
      mask prompts: str "dref"
  wires:
  Constant/1 -> Subsystem/1(value)

== system UNIFIER1/C7A_HARW/Aero/AlphaVtail ==
  V_w (m/s) : Inport
  omega_w (rad/s) : Inport  Port=2
  xyz_nodes (m) : Inport  Port=3  Partition=on  PartitionDimension=2  PartitionWidth=1  PartitionOffset=0
  3x3 Cross Product : sharedutil/3x3 Cross Product  aMode=aMode
  Asin : Trigonometry  Operator=asin
  Atan : Trigonometry  Operator=atan
  Cast : DataTypeConversion  OutDataTypeStr=single  SaturateOnIntegerOverflow=off  RndMeth=Floor
  Constant : Constant  Value=xyz_cg
  Constant1 : Constant  Value=eps  OutDataTypeStr=single
  Demux : Demux  Outputs=3
  Divide : Product  Inputs=*/
  Divide1 : Product  Inputs=*/
  For Each : ForEach  DisableCoverage=on  SpecifiedNumIters=16
  Mux : Mux  Inputs=3
  Sum : Sum  Inputs=+-
  Sum1 : Sum  Inputs=++|
  Sum2 : Sum  Inputs=|++
  Sum3 : Sum  Inputs=|++
  V_inf : Fcn  Expr=sqrt(u(1)^2+u(2)^2+u(3)^2)
  alpha_nodes : Outport  ConcatenationDimension=2
  beta_nodes : Outport  Port=2  ConcatenationDimension=2
  V_nodes : Outport  Port=3  ConcatenationDimension=2
  wires:
  3x3 Cross Product/1 -> Sum1/1
  Sum/1 -> 3x3 Cross Product/1
  Constant/1 -> Cast/1
  xyz_nodes (m)/1 -> Sum/2
  omega_w (rad/s)/1 -> 3x3 Cross Product/2
  V_w (m/s)/1 -> Sum1/2
  Sum1/1 -> Demux/1
  Demux/1 -> Sum2/1, Mux/1  "u"
  Demux/3 -> Mux/3, Divide/1  "w"
  Divide/1 -> Atan/1
  Atan/1 -> alpha_nodes/1
  Sum2/1 -> Divide/2
  Constant1/1 -> Sum3/2, Sum2/2
  Divide1/1 -> Asin/1
  Demux/2 -> Mux/2, Divide1/1
  Mux/1 -> V_inf/1
  Asin/1 -> beta_nodes/1  "beta"
  V_inf/1 -> Sum3/1
  Sum3/1 -> V_nodes/1, Divide1/2
  Cast/1 -> Sum/1

== system UNIFIER1/C7A_HARW/Aero/AlphaWIng ==
  V_w (m/s) : Inport
  omega_w (rad/s) : Inport  Port=2
  xyz_nodes (m) : Inport  Port=3  Partition=on  PartitionDimension=2  PartitionWidth=1  PartitionOffset=0
  Cast : DataTypeConversion  OutDataTypeStr=single  SaturateOnIntegerOverflow=off  RndMeth=Floor
  ComputeAlphaBetaV : Subsystem
  Constant : Constant  Value=xyz_cg
  Cross Product : matrix_library/Cross Product
  For Each : ForEach  DisableCoverage=on  SpecifiedNumIters=14
  Sum : Sum  Inputs=+-
  Sum1 : Sum  Inputs=++|
  Terminator : Terminator
  alpha_nodes : Outport  ConcatenationDimension=2
  V_nodes : Outport  Port=2  ConcatenationDimension=2
  wires:
  Cross Product/1 -> Sum1/1
  Sum/1 -> Cross Product/1
  Constant/1 -> Cast/1
  xyz_nodes (m)/1 -> Sum/2
  omega_w (rad/s)/1 -> Cross Product/2
  V_w (m/s)/1 -> Sum1/2
  Cast/1 -> Sum/1
  Sum1/1 -> ComputeAlphaBetaV/1(V_w_local)
  ComputeAlphaBetaV/3(V_nodes) -> V_nodes/1
  ComputeAlphaBetaV/2(beta_nodes) -> Terminator/1
  ComputeAlphaBetaV/1(alpha_nodes) -> alpha_nodes/1

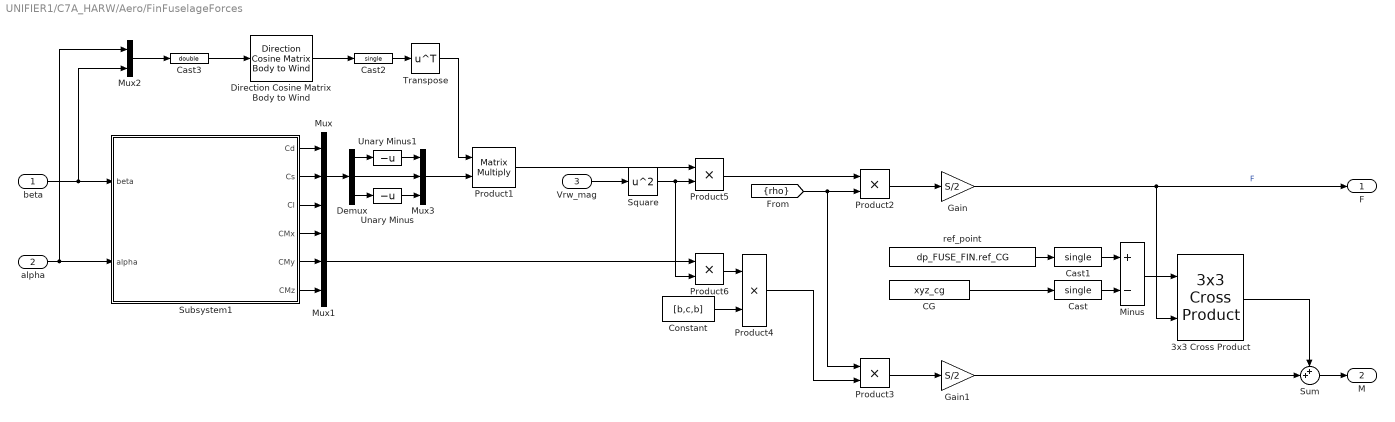
== system UNIFIER1/C7A_HARW/Aero/FinFuselageForces ==
  beta : Inport
  alpha : Inport  Port=2
  Vrw_mag : Inport  Port=3  OutDataTypeStr=single
  3x3 Cross Product : sharedutil/3x3 Cross Product  aMode=aMode
  CG : Constant  Value=xyz_cg
  Cast : DataTypeConversion  OutDataTypeStr=single  SaturateOnIntegerOverflow=off  RndMeth=Floor
  Cast1 : DataTypeConversion  OutDataTypeStr=single  SaturateOnIntegerOverflow=off  RndMeth=Floor
  Cast2 : DataTypeConversion  OutDataTypeStr=single  SaturateOnIntegerOverflow=off  RndMeth=Floor
  Cast3 : DataTypeConversion  OutDataTypeStr=double  SaturateOnIntegerOverflow=off  RndMeth=Floor
  Constant : Constant  Value=[b,c,b]
  Demux : Demux  Outputs=3
  Direction Cosine Matrix Body to Wind : aerolibtransform2/Direction Cosine Matrix Body to Wind
  Gain : Gain  Gain=S/2
  Gain1 : Gain  Gain=S/2
  Minus : Sum  Inputs=+-
  Mux : Mux  Inputs=3
  Mux1 : Mux  Inputs=3
  Mux2 : Mux  Inputs=2
  Mux3 : Mux  Inputs=3
  Product1 : Product  Multiplication=Matrix(*)
  Product{2..6} (5 alike) : Product
  Square : Math  Operator=square
  Subsystem1 : Subsystem
  Sum : Sum  Inputs=++|
  Transpose : Math  Operator=transpose
  Unary Minus : UnaryMinus
  Unary Minus1 : UnaryMinus
  ref_point : Constant  Value=dp_FUSE_FIN.ref_CG
  F : Outport
  M : Outport  Port=2
  wires:
  Mux/1 -> Demux/1
  Product6/1 -> Product4/1
  Mux1/1 -> Product6/1
  Product5/1 -> Product2/1
  Vrw_mag/1 -> Square/1
  Product1/1 -> Product5/1
  Square/1 -> Product5/2, Product6/2
  Unary Minus1/1 -> Mux3/1
  Unary Minus/1 -> Mux3/3
  Mux3/1 -> Product1/2
  Demux/3 -> Unary Minus/1
  Demux/2 -> Mux3/2
  Demux/1 -> Unary Minus1/1
  Cast2/1 -> Transpose/1
  Cast3/1 -> Direction Cosine Matrix Body to Wind/1
  Direction Cosine Matrix Body to Wind/1 -> Cast2/1
  Transpose/1 -> Product1/1
  Mux2/1 -> Cast3/1
  Sum/1 -> M/1
  alpha/1 -> Subsystem1/2(alpha), Mux2/1
  beta/1 -> Subsystem1/1(beta), Mux2/2
  Cast1/1 -> Minus/1
  CG/1 -> Cast/1
  Minus/1 -> 3x3 Cross Product/1
  Cast/1 -> Minus/2
  ref_point/1 -> Cast1/1
  3x3 Cross Product/1 -> Sum/1
  Subsystem1/6(CMz) -> Mux1/3
  Subsystem1/5(CMy) -> Mux1/2
  Subsystem1/4(CMx) -> Mux1/1
  Subsystem1/3(Cl) -> Mux/3
  Subsystem1/2(Cs) -> Mux/2
  Subsystem1/1(Cd) -> Mux/1
  Product3/1 -> Gain1/1
  Gain/1 -> 3x3 Cross Product/2, F/1  "F"
  Constant/1 -> Product4/2
  [rho] -> Product3/1, Product2/2
  Gain1/1 -> Sum/2
  Product4/1 -> Product3/2
  Product2/1 -> Gain/1

== system UNIFIER1/C7A_HARW/Aero/InducedAngleOfAttack ==
  flapL_defl : Inport
  flapR_defl : Inport  Port=2
  wing_alpha_nodes : Inport  Port=3  PortDimensions=14
  wing_V_nodes : Inport  Port=4  PortDimensions=14
  wing_DEP_J : Inport  Port=5  PortDimensions=12
  vtail_V_nodes : Inport  Port=6
  1-D Lookup Table : Lookup_n-D  NumberOfTableDimensions=1  BreakpointsForDimension1=wing_nodes(2,5:10)  BeginIndexSearchUsingPreviousIndexResult=on  TableSource=Input port  Table=tanh([-5:5])  ExtrapMethod=Clip  InternalRulePriority=Speed  RndMeth=Simplest
      settings: InputPortMap=u0,p221
  1-D Lookup Table1 : Lookup_n-D  NumberOfTableDimensions=1  BreakpointsForDimension1=wing_nodes(2,5:10)  BeginIndexSearchUsingPreviousIndexResult=on  TableSource=Input port  Table=tanh([-5:5])  ExtrapMethod=Clip  InternalRulePriority=Speed  RndMeth=Simplest
      settings: InputPortMap=u0,p221
  1-D Lookup Table2 : Lookup_n-D  NumberOfTableDimensions=1  BreakpointsForDimension1=wing_nodes(2,5:10)  BeginIndexSearchUsingPreviousIndexResult=on  TableSource=Input port  Table=tanh([-5:5])  ExtrapMethod=Clip  InternalRulePriority=Speed  RndMeth=Simplest
      settings: InputPortMap=u0,p221
  Constant : Constant  Value=ones(1,8)
  Constant1 : Constant  Value=ones(1,8)
  Constant7 : Constant  Value=vtail_nodes(2,:)
  Mux : Mux  Inputs=2
  Product : Product
  Product1 : Product
  Selector : Selector  InputPortWidth=14  IndexOptions=Index vector (dialog)  Indices=[5:10]  OutputSizes=1
  Selector1 : Selector  InputPortWidth=14  IndexOptions=Index vector (dialog)  Indices=[5:10]  OutputSizes=1
  Selector2 : Selector  InputPortWidth=12  IndexOptions=Index vector (dialog)  Indices=[4:9]  OutputSizes=1
  V_induced : Interpolation_n-D  NumberOfTableDimensions=5  Table=dp_VTAIL_INDUCED.V_induced  NumSelectionDims=1  InternalRulePriority=Speed  TableDataTypeStr=Inherit: Inherit from 'Table data'
      settings: InputPortMap=u0,u1,u2,u3,u4,u5,u6,u7,u8
  addDelay : Subsystem
  alpha_induced : Interpolation_n-D  NumberOfTableDimensions=5  Table=dp_VTAIL_INDUCED.alpha_induced  NumSelectionDims=1  InternalRulePriority=Speed  TableDataTypeStr=Inherit: Inherit from 'Table data'
      settings: InputPortMap=u0,u1,u2,u3,u4,u5,u6,u7,u8
  preLook : Subsystem
  vtail_alpha_induced_nodes : Outport  PortDimensions=16
  vtail_V_induced_nodes : Outport  Port=2  PortDimensions=16
  wires:
  1-D Lookup Table1/1 -> preLook/3(wing_V_inf)
  1-D Lookup Table2/1 -> preLook/4(wing_DEP_J)
  1-D Lookup Table/1 -> preLook/2(wing_alphas)
  Constant7/1 -> 1-D Lookup Table/1, 1-D Lookup Table2/1, 1-D Lookup Table1/1
  wing_V_nodes/1 -> Selector1/1
  wing_alpha_nodes/1 -> Selector/1
  preLook/1(Out1) -> alpha_induced/1, V_induced/1
  preLook/2(Out2) -> alpha_induced/2, V_induced/2
  preLook/3(Out8) -> alpha_induced/3, V_induced/3
  preLook/4(Out9) -> alpha_induced/4, V_induced/4
  preLook/5(Out3) -> alpha_induced/5, V_induced/5
  preLook/6(Out4) -> alpha_induced/6, V_induced/6
  preLook/7(Out6) -> alpha_induced/7, V_induced/7
  preLook/8(Out7) -> alpha_induced/8, V_induced/8
  preLook/9(Out5) -> alpha_induced/9, V_induced/9
  wing_DEP_J/1 -> Selector2/1
  flapL_defl/1 -> Product/2
  Constant/1 -> Product/1
  Constant1/1 -> Product1/1
  flapR_defl/1 -> Product1/2
  Product/1 -> Mux/1
  Product1/1 -> Mux/2
  Mux/1 -> preLook/1(wing_flap_defl)
  V_induced/1 -> addDelay/1(V_induced)
  addDelay/1(V_delayed) -> vtail_V_induced_nodes/1
  addDelay/2(alpha_delayed) -> vtail_alpha_induced_nodes/1
  vtail_V_nodes/1 -> addDelay/3(vtail_V_nodes)
  alpha_induced/1 -> addDelay/2(alpha_induced)
  Selector/1 -> 1-D Lookup Table/2
  Selector1/1 -> 1-D Lookup Table1/2
  Selector2/1 -> 1-D Lookup Table2/2

== system UNIFIER1/C7A_HARW/Aero/VtailForces ==
  alpha_nodes : Inport  PortDimensions=16
  beta_nodes : Inport  Port=2  PortDimensions=16
  V_nodes : Inport  Port=3  PortDimensions=16
  rudeL_defl : Inport  Port=4
  rudeR_defl : Inport  Port=5
  Constant : Constant  Value=ones(1,8)
  Constant1 : Constant  Value=ones(1,8)
  Matrix Concatenate1 : Concatenate  NumInputs=3  Mode=Multidimensional array  ConcatenateDimension=2
  Matrix Concatenate2 : Concatenate  NumInputs=3  Mode=Multidimensional array  ConcatenateDimension=2
  Mux : Mux  Inputs=2
  Product : Product
  Product1 : Product
  Reshape : Reshape
  Reshape1 : Reshape
  Subsystem : Subsystem
  Transpose : Math  Operator=transpose
  Transpose1 : Math  Operator=transpose
  VtailForces : Subsystem
  F : Outport
  M : Outport  Port=2
  wires:
  alpha_nodes/1 -> VtailForces/2(alpha_nodes)
  beta_nodes/1 -> VtailForces/3(beta_nodes)
  Product/1 -> Mux/1
  Product1/1 -> Mux/2
  Mux/1 -> VtailForces/1(rude_defl_nodes)
  Constant1/1 -> Product1/1
  Constant/1 -> Product/1
  rudeL_defl/1 -> Product/2
  rudeR_defl/1 -> Product1/2
  VtailForces/4(CMx) -> Matrix Concatenate2/1  "CMx"
  VtailForces/6(CMz) -> Matrix Concatenate2/3  "CMz"
  Matrix Concatenate2/1 -> Transpose1/1
  Subsystem/2(M) -> Reshape/1
  Transpose/1 -> Subsystem/2(F_matrix)
  Transpose1/1 -> Subsystem/3(M_matrix)
  VtailForces/2(Cy) -> Matrix Concatenate1/2  "CFy"
  VtailForces/5(CMy) -> Matrix Concatenate2/2  "CMy"
  VtailForces/1(Cx) -> Matrix Concatenate1/1  "CFx"
  Matrix Concatenate1/1 -> Transpose/1
  Subsystem/1(F) -> Reshape1/1
  VtailForces/3(Cz) -> Matrix Concatenate1/3  "CFz"
  V_nodes/1 -> Subsystem/1(V_nodes)
  Reshape/1 -> M/1
  Reshape1/1 -> F/1

== system UNIFIER1/C7A_HARW/Aero/WingForces ==
  flapL_defl : Inport
  flapR_defl : Inport  Port=2
  ailL_defl : Inport  Port=3
  ailR_defl : Inport  Port=4
  DEP_J : Inport  Port=5  PortDimensions=12
  alpha_nodes : Inport  Port=6  PortDimensions=14
  V_node : Inport  Port=7  PortDimensions=14
  Demux : Demux  Outputs=3
  Demux1 : Demux  Outputs=3
  Left : Subsystem
  Mux : Mux  Inputs=3
  Mux1 : Mux  Inputs=3
  Reshape : Reshape
  Reshape1 : Reshape
  Right : Subsystem
  Subsystem : Subsystem
  Sum : Sum  Inputs=|++
  Sum1 : Sum  Inputs=|++
  Unary Minus : UnaryMinus
  Unary Minus1 : UnaryMinus
  Unary Minus2 : UnaryMinus
  F : Outport
  M : Outport  Port=2
  wires:
  ailL_defl/1 -> Left/2(aile_defl)
  flapL_defl/1 -> Left/1(flap_defl)
  ailR_defl/1 -> Right/2(aile_defl)
  DEP_J/1 -> Subsystem/1(DEP_J)
  flapR_defl/1 -> Right/1(flap_defl)
  alpha_nodes/1 -> Subsystem/2(alpha_nodes)
  V_node/1 -> Subsystem/3(V_nodes)
  Subsystem/1(DEP_J_Left) -> Left/3(DEP_J)
  Subsystem/2(alpha_nodes_Left) -> Left/4(alpha)
  Subsystem/3(V_nodes_Left) -> Left/5(V_node)
  Left/1(F) -> Demux/1
  Left/2(M) -> Demux1/1
  Demux/2 -> Unary Minus/1
  Demux1/1 -> Unary Minus1/1
  Demux1/3 -> Unary Minus2/1
  Demux1/2 -> Mux/2
  Unary Minus1/1 -> Mux/1
  Unary Minus2/1 -> Mux/3
  Unary Minus/1 -> Mux1/2
  Demux/1 -> Mux1/1
  Demux/3 -> Mux1/3
  Mux1/1 -> Sum/1
  Sum/1 -> F/1
  Mux/1 -> Sum1/1
  Sum1/1 -> M/1
  Right/1(F) -> Reshape/1
  Right/2(M) -> Reshape1/1
  Subsystem/5(alpha_nodes_Right) -> Right/4(alpha)
  Subsystem/6(V_nodes_Right) -> Right/5(V_node)
  Subsystem/4(DEP_J_Right) -> Right/3(DEP_J)
  Reshape/1 -> Sum/2
  Reshape1/1 -> Sum1/2

== system UNIFIER1/C7A_HARW/Aero/additionalDrag ==
  note: Landing gear drag:
      | Loftin Jr, L. K. (1980). Subsonic aircraft: Evolution and the matching of size to performance (No. L-13367).
  note: Wing mounted nacelles:
      | (Estimate using OpenVSP - Jenkinson Wing Mounted Nacelle)
      | =6*0.00043=0.00258
      | + cooling drag of 0.015
  alpha (rad) : Inport
  beta (rad) : Inport  Port=2
  Vrw_mag : Inport  Port=3
  rho (kg/m^3) : Inport  Port=4
  u4 (gear) : Inport  Port=5
  Cast : DataTypeConversion  OutDataTypeStr=single  SaturateOnIntegerOverflow=off  RndMeth=Floor
  Cast1 : DataTypeConversion  OutDataTypeStr=single  SaturateOnIntegerOverflow=off  RndMeth=Floor
  Cast2 : DataTypeConversion  OutDataTypeStr=double  SaturateOnIntegerOverflow=off  RndMeth=Floor
  Constant1 : Constant  Value=0  OutDataTypeStr=single
  Direction Cosine Matrix Body to Wind : aerolibtransform2/Direction Cosine Matrix Body to Wind
  Gain : Gain  Gain=S/2
  Math Function : Math  Operator=square
  Mux : Mux  Inputs=2
  Mux1 : Mux  Inputs=3
  Product : Product  OutDataTypeStr=single
  Product1 : Product  Multiplication=Matrix(*)
  Product2 : Product
  Product3 : Product
  Sum : Sum  Inputs=|++
  Transpose : Math  Operator=transpose
  Unary Minus : UnaryMinus
  extra_drag : Constant  Value=0.00258+0.015  OutDataTypeStr=single
  gear_drag : Constant  Value=0.015  OutDataTypeStr=single
  F_additional : Outport
  wires:
  alpha (rad)/1 -> Mux/1
  Math Function/1 -> Product/2
  Product/1 -> Unary Minus/1
  Gain/1 -> Product/1
  Product2/1 -> Gain/1
  extra_drag/1 -> Sum/1
  Vrw_mag/1 -> Math Function/1
  rho (kg/m^3)/1 -> Product2/2
  Direction Cosine Matrix Body to Wind/1 -> Cast1/1
  Mux/1 -> Cast2/1
  beta (rad)/1 -> Mux/2
  Unary Minus/1 -> Mux1/1
  Transpose/1 -> Product1/1
  Mux1/1 -> Product1/2
  Constant1/1 -> Mux1/2, Mux1/3
  Product1/1 -> Cast/1
  Cast/1 -> F_additional/1
  Cast1/1 -> Transpose/1
  Cast2/1 -> Direction Cosine Matrix Body to Wind/1
  u4 (gear)/1 -> Product3/2
  gear_drag/1 -> Product3/1
  Sum/1 -> Product2/1
  Product3/1 -> Sum/2
